simulink model "FitValidation"  (R2018a)
settings: Solver=VariableStepAuto  StartTime=0.0  StopTime=1  MaxStep=1e-4  RelTol=1e-3
values from neighbouring files (symbols this model uses):
  C1 = 22e-6    (= 2.2e-05)    [SimulinkInit.m]
undefined symbols (not defined in the file or in its folder): A1, B, ss1
settings Model: Creator=erich  LastModifiedBy=MarioAndres
settings CodeAppCC: StateflowObjectComments=on

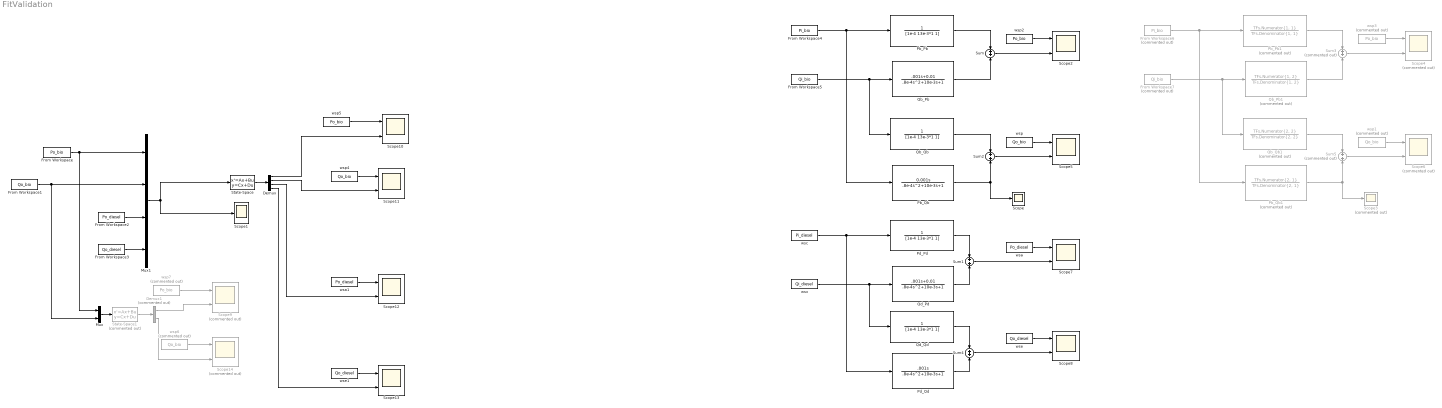
== system FitValidation ==
  Demux : Demux
  Demux1 : Demux  Commented=on  Outputs=2
  From Workspace : FromWorkspace  VariableName=Po_bio  SampleTime=0
  From Workspace1 : FromWorkspace  VariableName=Qo_bio  SampleTime=0
  From Workspace2 : FromWorkspace  VariableName=Po_diesel  SampleTime=0
  From Workspace3 : FromWorkspace  VariableName=Qo_diesel  SampleTime=0
  From Workspace4 : FromWorkspace  VariableName=Pi_bio  SampleTime=0
  From Workspace5 : FromWorkspace  VariableName=Qi_bio  SampleTime=0
  From Workspace6 : FromWorkspace  Commented=on  VariableName=Pi_bio  SampleTime=0
  From Workspace7 : FromWorkspace  Commented=on  VariableName=Qi_bio  SampleTime=0
  Mux : Mux  Inputs=2
  Mux1 : Mux
  Pb_Pb : TransferFcn  Denominator=[1e-4 13e-3*1 1]
  Pb_Pb1 : TransferFcn  Commented=on  Numerator=TFs.Numerator{1, 1}  Denominator=TFs.Denominator{1, 1}
  Pb_Qb : TransferFcn  Numerator=[0.001 0]  Denominator=[.8e-4 10e-3 1]
  Pb_Qb1 : TransferFcn  Commented=on  Numerator=TFs.Numerator{2, 1}  Denominator=TFs.Denominator{2, 1}
  Pd_Pd : TransferFcn  Denominator=[1e-4 13e-3*1 1]
  Pd_Qd : TransferFcn  Numerator=[.001 0]  Denominator=[.8e-4 10e-3 1]
  Qb_Pb : TransferFcn  Numerator=[.001 0.01]  Denominator=[.8e-4 10e-3 1]
  Qb_Pb1 : TransferFcn  Commented=on  Numerator=TFs.Numerator{1, 2}  Denominator=TFs.Denominator{1, 2}
  Qb_Qb : TransferFcn  Denominator=[1e-4 13e-3*1 1]
  Qb_Qb1 : TransferFcn  Commented=on  Numerator=TFs.Numerator{2, 2}  Denominator=TFs.Denominator{2, 2}
  Qd_Pd : TransferFcn  Numerator=[.001 0.01]  Denominator=[.8e-4 10e-3 1]
  Qd_Qd : TransferFcn  Denominator=[1e-4 13e-3*1 1]
  Scope : Scope
  Scope1 : Scope
  Scope{2,5,7..8,10..13} (8 alike) : Scope  NumInputPorts=2
  Scope{4,6,9,14} (4 alike) : Scope  Commented=on  NumInputPorts=2
  Scope3 : Scope  Commented=on
  State-Space : StateSpace  A=ss1.A  B=ss1.B  C=ss1.C  D=ss1.D  InitialCondition=0
  State-Space1 : StateSpace  Commented=on  A=A1  B=B  C=C1  D=zeros(2,2)  InitialCondition=0
  Sum{,1..2,4} (4 alike) : Sum  Inputs=+|+
  Sum3 : Sum  Commented=on  Inputs=+|+
  Sum5 : Sum  Commented=on  Inputs=+|+
  wsa : FromWorkspace  VariableName=Po_diesel  SampleTime=0
  wsa1 : FromWorkspace  VariableName=Po_diesel  SampleTime=0
  wsc : FromWorkspace  VariableName=Pi_diesel  SampleTime=0
  wse : FromWorkspace  VariableName=Qo_diesel  SampleTime=0
  wse1 : FromWorkspace  VariableName=Qo_diesel  SampleTime=0
  wsp : FromWorkspace  VariableName=Qo_bio  SampleTime=0
  wsp1 : FromWorkspace  Commented=on  VariableName=Qo_bio  SampleTime=0
  wsp2 : FromWorkspace  VariableName=Po_bio  SampleTime=0
  wsp3 : FromWorkspace  Commented=on  VariableName=Po_bio  SampleTime=0
  wsp4 : FromWorkspace  VariableName=Qo_bio  SampleTime=0
  wsp5 : FromWorkspace  VariableName=Po_bio  SampleTime=0
  wsp6 : FromWorkspace  Commented=on  VariableName=Qo_bio  SampleTime=0
  wsp7 : FromWorkspace  Commented=on  VariableName=Po_bio  SampleTime=0
  wsx : FromWorkspace  VariableName=Qi_diesel  SampleTime=0
  wires:
  From Workspace3/1 -> Mux1/4
  From Workspace2/1 -> Mux1/3
  From Workspace1/1 -> Mux/2, Mux1/2
  From Workspace/1 -> Mux/1, Mux1/1
  Mux1/1 -> State-Space/1, Scope1/1
  wsp2/1 -> Scope2/1
  Sum/1 -> Scope2/2
  Pb_Pb/1 -> Sum/1
  Qb_Pb/1 -> Sum/2
  Pb_Qb/1 -> Sum2/2, Scope/1
  Qb_Qb/1 -> Sum2/1
  Sum2/1 -> Scope5/2
  wsp/1 -> Scope5/1
  From Workspace5/1 -> Qb_Qb/1, Qb_Pb/1
  From Workspace4/1 -> Pb_Qb/1, Pb_Pb/1
  wsc/1 -> Pd_Pd/1, Pd_Qd/1
  wsx/1 -> Qd_Pd/1, Qd_Qd/1
  wse/1 -> Scope8/1
  Sum4/1 -> Scope8/2
  Qd_Qd/1 -> Sum4/1
  Pd_Qd/1 -> Sum4/2
  Qd_Pd/1 -> Sum1/2
  Pd_Pd/1 -> Sum1/1
  Sum1/1 -> Scope7/2
  wsa/1 -> Scope7/1
  From Workspace6/1 -> Pb_Pb1/1, Pb_Qb1/1
  From Workspace7/1 -> Qb_Pb1/1, Qb_Qb1/1
  wsp1/1 -> Scope6/1
  Sum5/1 -> Scope6/2
  Qb_Qb1/1 -> Sum5/1
  Pb_Qb1/1 -> Scope3/1, Sum5/2
  Qb_Pb1/1 -> Sum3/2
  Pb_Pb1/1 -> Sum3/1
  Sum3/1 -> Scope4/2
  wsp3/1 -> Scope4/1
  wse1/1 -> Scope13/1
  wsp5/1 -> Scope10/1
  wsp4/1 -> Scope11/1
  wsa1/1 -> Scope12/1
  State-Space/1 -> Demux/1
  Demux/1 -> Scope10/2
  Demux/2 -> Scope11/2
  Demux/3 -> Scope12/2
  Demux/4 -> Scope13/2
  Mux/1 -> State-Space1/1
  wsp6/1 -> Scope14/1
  wsp7/1 -> Scope9/1
  State-Space1/1 -> Demux1/1
  Demux1/1 -> Scope9/2
  Demux1/2 -> Scope14/2
